simulink model "Lab1ex3"  (R2020a)
settings: Solver=VariableStepAuto  StartTime=0.0  StopTime=120  RelTol=1e-3
settings Model: Creator=ariana  LastModifiedBy=ariana

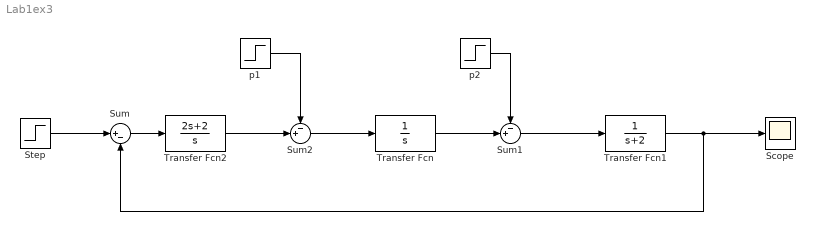
== system Lab1ex3 ==
  Scope : Scope
  Step : Step  SampleTime=0
  Sum : Sum  Inputs=|+-
  Sum1 : Sum  Inputs=-+|
  Sum2 : Sum  Inputs=-+|
  Transfer Fcn : TransferFcn  Denominator=[1 0]
  Transfer Fcn1 : TransferFcn  Denominator=[1 2]
  Transfer Fcn2 : TransferFcn  Numerator=[2 2]  Denominator=[1 0]
  p1 : Step  Time=30  SampleTime=0
  p2 : Step  Time=60  SampleTime=0
  wires:
  Transfer Fcn1/1 -> Sum/2, Scope/1
  Sum2/1 -> Transfer Fcn/1
  Transfer Fcn/1 -> Sum1/2
  Sum1/1 -> Transfer Fcn1/1
  Step/1 -> Sum/1
  p1/1 -> Sum2/1
  p2/1 -> Sum1/1
  Sum/1 -> Transfer Fcn2/1
  Transfer Fcn2/1 -> Sum2/2
